simulink subsystem "POWER"  (R2025b)
settings: Solver=VariableStepAuto  StartTime=0.0  StopTime=10.0  RelTol=1e-3
settings Model: Creator=JesseJabezArendse  LastModifiedBy=JesseJabezArendse

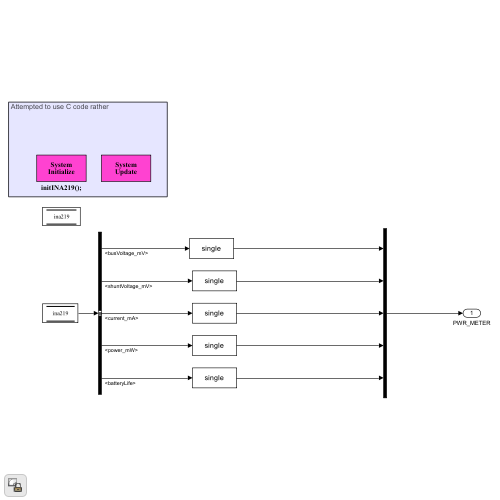
[thumbnail: Simulink's stored preview of the top-level diagram]
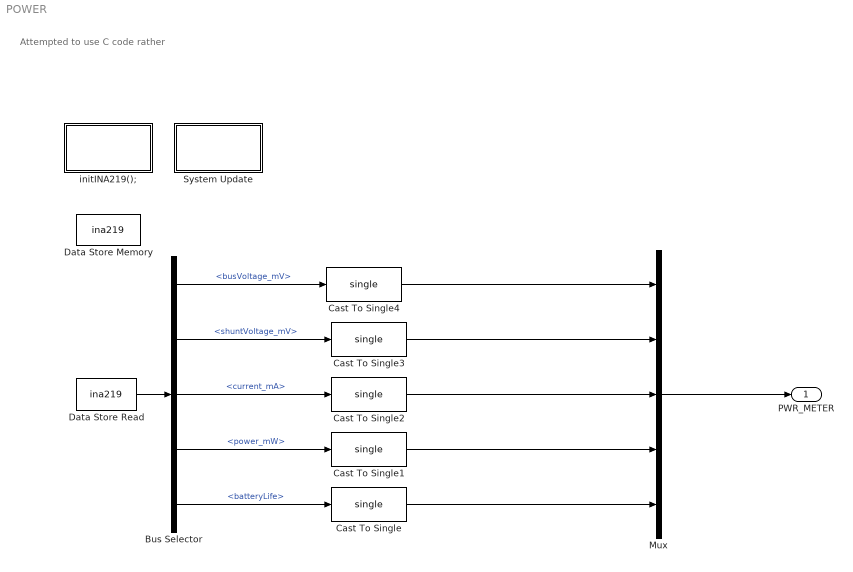
== system POWER ==
  note: Attempted to use C code rather
  Bus Selector : BusSelector  OutputSignals=busVoltage_mV,shuntVoltage_mV,current_mA,power_mW,batteryLife
  Cast To Single{,1..4} (5 alike) : DataTypeConversion  OutDataTypeStr=single  SaturateOnIntegerOverflow=off  RndMeth=Floor
  Data Store Memory : DataStoreMemory  DataStoreName=ina219  WriteAfterWriteMsg=warning  ShowAdditionalParam=off  OutDataTypeStr=Bus: INA219_t
  Data Store Read : DataStoreRead  DataStoreName=ina219  IndexOptions=Index vector (dialog)  Indices=1  OutputSizes=1
  Mux : Mux  Inputs=5
  System Update : Subsystem  mask(System Update){ShowInLibBrowser=0}
      mask prompts: ShowInLibBrowser "Simulink:masks:CustCodeMaskParam1_MP"
      settings: CopyFcn=cccopyfcn(gcb)  OpenFcn=ccopenfcn('System Update Function')
      mask Help: eval('feval(''rtwprivate'',''rtwhelpview'',''rtw_sys_update_block'')');
      mask Display: disp('System\nUpdate');
  initINA219(); : Subsystem  mask(System Initialize){ShowInLibBrowser=0}
      mask prompts: ShowInLibBrowser "Simulink:masks:CustCodeMaskParam1_MP"
      settings: CopyFcn=cccopyfcn(gcb)  OpenFcn=ccopenfcn('System Initialize Function')
      mask Help: eval('feval(''rtwprivate'',''rtwhelpview'',''rtw_sys_initialize_block'')');
      mask Display: disp('System\nInitialize');
  PWR_METER : Outport
  wires:
  Bus Selector/1 -> Cast To Single4/1  "<busVoltage_mV>"
  Bus Selector/5 -> Cast To Single/1  "<batteryLife>"
  Cast To Single2/1 -> Mux/3
  Cast To Single1/1 -> Mux/4
  Cast To Single3/1 -> Mux/2
  Cast To Single/1 -> Mux/5
  Cast To Single4/1 -> Mux/1
  Bus Selector/3 -> Cast To Single2/1  "<current_mA>"
  Bus Selector/4 -> Cast To Single1/1  "<power_mW>"
  Mux/1 -> PWR_METER/1
  Data Store Read/1 -> Bus Selector/1
  Bus Selector/2 -> Cast To Single3/1  "<shuntVoltage_mV>"

== system POWER/System Update ==

== system POWER/initINA219(); ==
